simulink model "genpath_user_iface_dc"  (R2022a)
settings: Solver=FixedStepDiscrete  StartTime=0.0  StopTime=inf  RelTol=1e-3  EnableMultiTasking=on
undefined symbols (not defined in the file or in its folder): HW_LOG_VEC_SIZE, HW_LS, HW_RS
libraries: mcbcontrolslib x4, instrumentseriallib x3
settings Model: SimulationMode=accelerator  Creator=61301765  LastModifiedBy=61301765
settings OptimizationCC: DefaultParameterBehavior=Inlined  DefaultUnderspecifiedDataType=single  EnhancedBackFolding=on  PassReuseOutputArgsAs=Individual arguments  ZeroExternalMemoryAtStartup=off  MaxStackSize=64  OptimizeBlockOrder=speed  DifferentSizesBufferReuse=on  OptimizationCustomize=off  EfficientTunableParamExpr=on
settings DebuggingCC: ParameterTunabilityLossMsg=error  UnconnectedInputMsg=warning  UnconnectedOutputMsg=warning  UnconnectedLineMsg=warning
settings HardwareCC: ProdBitPerChar=16  ProdBitPerInt=16  ProdBitPerPointer=32  ProdBitPerSizeT=32  ProdBitPerPtrDiffT=32  ProdLargestAtomicInteger=Integer  ProdLargestAtomicFloat=None  ProdWordSize=16  ProdLongLongMode=on  ProdHWDeviceType=Texas Instruments->C2000
settings SFSimCC: MATLABDynamicMemAlloc=off
settings RTWCC: SystemTargetFile=ert.tlc  TemplateMakefile=ert_default_tmf  Toolchain=Texas Instruments Code Composer Studio (C2000)  DLArmComputeVersion=19.05
settings CodeAppCC: ForceParamTrailComments=on  IgnoreCustomStorageClasses=off  OperatorAnnotations=on  SimulinkDataObjDesc=on  SFDataObjDesc=on  InsertBlockDesc=on
settings ERTTargetCC: ExtModeStaticAllocSize=5000  ERTCustomFileTemplate=example_file_process.tlc

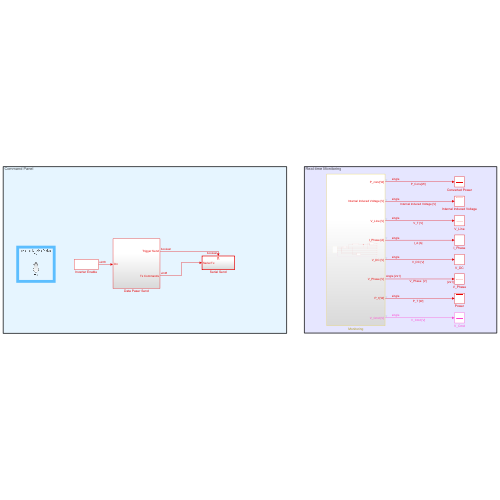
[thumbnail: Simulink's stored preview of the top-level diagram]
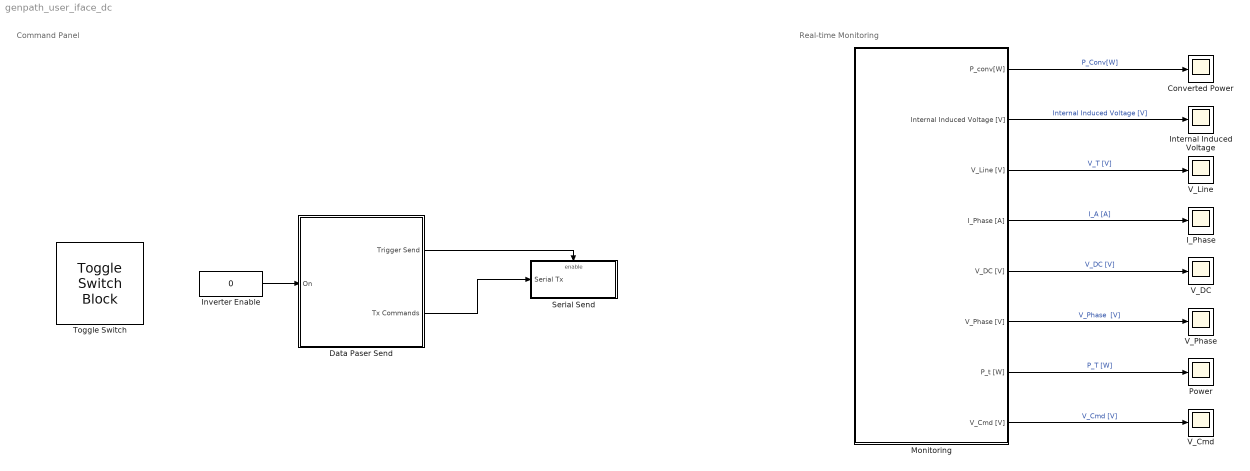
== system genpath_user_iface_dc ==
  note: Real-time Monitoring
  note: Command Panel
  Converted Power : Scope
  Data Paser Send : Subsystem
  I_Phase : Scope
  Internal Induced Voltage : Scope
  Inverter Enable : Constant  Value=0  VectorParams1D=off  OutDataTypeStr=uint8  SampleTime=-1
  Monitoring : Subsystem
  Power : Scope
  Serial Send : Subsystem  TreatAsAtomicUnit=on
  Toggle Switch : ToggleSwitchBlock
      settings: Values={{'Off', 'On'}, [0 1]}
  V_Cmd : Scope
  V_DC : Scope
  V_Line : Scope
  V_Phase : Scope
  wires:
  Data Paser Send/2(Tx Commands) -> Serial Send/1(Serial Tx)
  Data Paser Send/1(Trigger Send) -> Serial Send/Enable
  Inverter Enable/1 -> Data Paser Send/1(On)
  Monitoring/1(P_conv[W]) -> Converted Power/1  "P_Conv[W]"
  Monitoring/3(V_Line [V]) -> V_Line/1  "V_T [V]"
  Monitoring/4(I_Phase [A]) -> I_Phase/1  "I_A [A]"
  Monitoring/5(V_DC [V]) -> V_DC/1  "V_DC [V]"
  Monitoring/6(V_Phase [V]) -> V_Phase/1  "V_Phase  [V]"
  Monitoring/7(P_t [W]) -> Power/1  "P_T [W]"
  Monitoring/2(Internal Induced Voltage [V]) -> Internal Induced Voltage/1  "Internal Induced Voltage [V]"
  Monitoring/8(V_Cmd [V]) -> V_Cmd/1  "V_Cmd [V]"

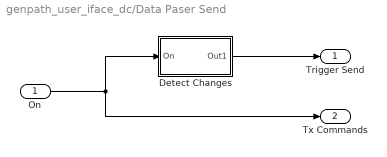
== system genpath_user_iface_dc/Data Paser Send ==
  On : Inport
  Detect Changes : Subsystem
  Trigger Send : Outport  VectorParamsAs1DForOutWhenUnconnected=off
  Tx Commands : Outport  Port=2  VectorParamsAs1DForOutWhenUnconnected=off
  wires:
  Detect Changes/1(Out1) -> Trigger Send/1
  On/1 -> Detect Changes/1(On), Tx Commands/1

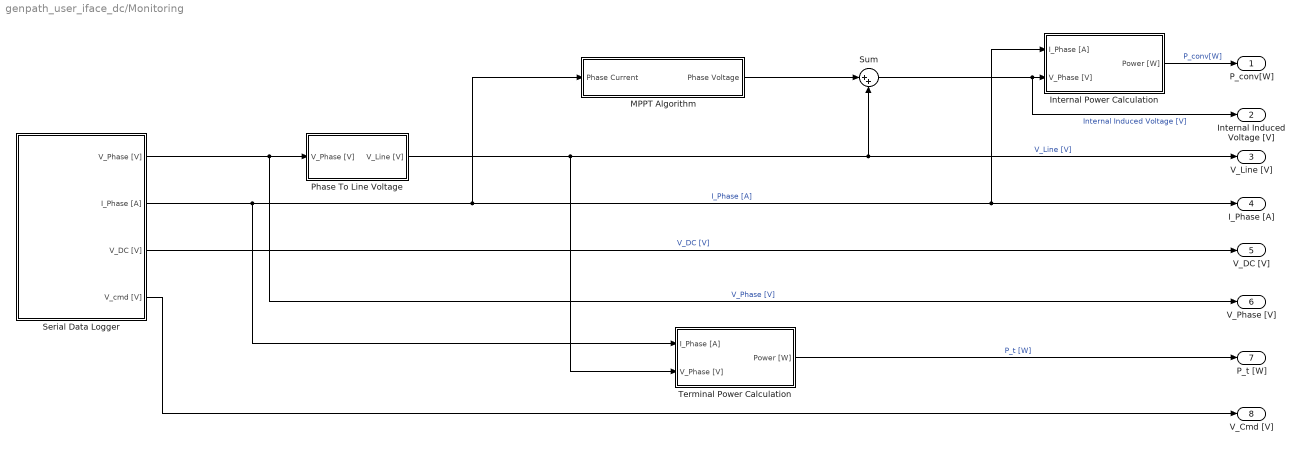
== system genpath_user_iface_dc/Monitoring ==
  Internal Power Calculation : Subsystem
  MPPT Algorithm : Subsystem
  Phase To Line Voltage : Subsystem
  Serial Data Logger : Subsystem
  Sum : Sum  Inputs=|++
  Terminal Power Calculation : Subsystem
  P_conv[W] : Outport
  Internal Induced Voltage [V] : Outport  Port=2
  V_Line [V] : Outport  Port=3
  I_Phase [A] : Outport  Port=4
  V_DC [V] : Outport  Port=5
  V_Phase [V] : Outport  Port=6
  P_t [W] : Outport  Port=7
  V_Cmd [V] : Outport  Port=8
  wires:
  Terminal Power Calculation/1(Power [W]) -> P_t [W]/1  "P_t [W]"
  Serial Data Logger/2(I_Phase [A]) -> Terminal Power Calculation/1(I_Phase [A]), MPPT Algorithm/1(Phase Current), I_Phase [A]/1, Internal Power Calculation/1(I_Phase [A])  "I_Phase [A]"
  Serial Data Logger/1(V_Phase [V]) -> V_Phase [V]/1, Phase To Line Voltage/1(V_Phase [V])  "V_Phase [V]"
  Phase To Line Voltage/1(V_Line [V]) -> Terminal Power Calculation/2(V_Phase [V]), Sum/2, V_Line [V]/1  "V_Line [V]"
  Serial Data Logger/3(V_DC [V]) -> V_DC [V]/1  "V_DC [V]"
  Sum/1 -> Internal Power Calculation/2(V_Phase [V]), Internal Induced Voltage [V]/1  "Internal Induced Voltage [V]"
  Internal Power Calculation/1(Power [W]) -> P_conv[W]/1  "P_conv[W]"
  Serial Data Logger/4(V_cmd [V]) -> V_Cmd [V]/1
  MPPT Algorithm/1(Phase Voltage) -> Sum/1

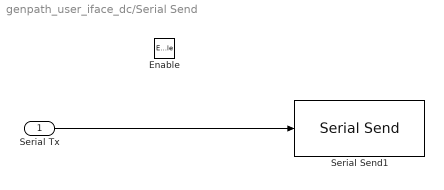
== system genpath_user_iface_dc/Serial Send ==
  Serial Tx : Inport
  Enable : EnablePort
  Serial Send1 : instrumentseriallib/Serial Send  PortSel=COM8  Port=COM8  ComPort=COM8  Header=[ 83 ]  Terminator=Custom terminator  CustomTerminator=[ 69 ]  EnableBlockingMode=on  SimulateUsing=Interpreted execution  BlockInModel=on  aMode=1
      settings: SourceProductBaseCode=OT,IC,MT
  wires:
  Serial Tx/1 -> Serial Send1/1

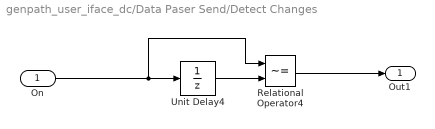
== system genpath_user_iface_dc/Data Paser Send/Detect Changes ==
  On : Inport
  Relational Operator4 : RelationalOperator  Operator=~=  OutDataTypeStr=boolean  InputSameDT=off
  Unit Delay4 : UnitDelay  SampleTime=-1  HasFrameUpgradeWarning=on
  Out1 : Outport  VectorParamsAs1DForOutWhenUnconnected=off
  wires:
  Unit Delay4/1 -> Relational Operator4/2
  On/1 -> Relational Operator4/1, Unit Delay4/1
  Relational Operator4/1 -> Out1/1

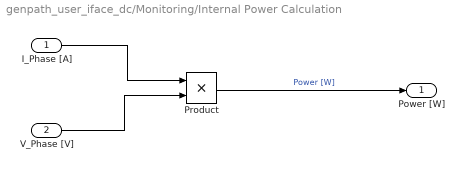
== system genpath_user_iface_dc/Monitoring/Internal Power Calculation ==
  I_Phase [A] : Inport
  V_Phase [V] : Inport  Port=2
  Product : Product
  Power [W] : Outport
  wires:
  Product/1 -> Power [W]/1  "Power [W]"
  V_Phase [V]/1 -> Product/2
  I_Phase [A]/1 -> Product/1

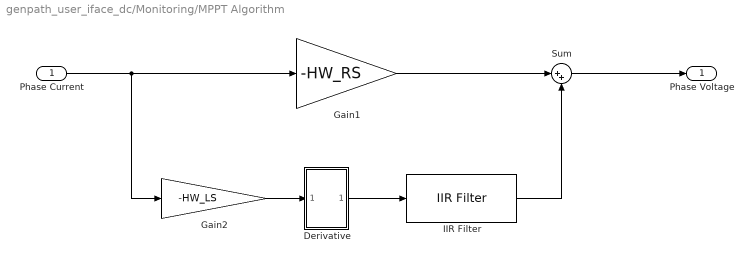
== system genpath_user_iface_dc/Monitoring/MPPT Algorithm ==
  Phase Current : Inport
  Derivative : Subsystem
  Gain1 : Gain  Gain=-HW_RS
  Gain2 : Gain  Gain=-HW_LS
  IIR Filter : mcbcontrolslib/IIR Filter  VariantControl=Low Pass Filter  VariantSelect=Low-pass  Filter_constant=0.2  advancedSettings=on  Ts=100e-6  cutOff_freq=397.8874
      settings: SourceProductBaseCode=MT
  Sum : Sum  Inputs=|++
  Phase Voltage : Outport
  wires:
  Phase Current/1 -> Gain2/1, Gain1/1
  Gain1/1 -> Sum/1
  IIR Filter/1 -> Sum/2
  Gain2/1 -> Derivative/1(In3)
  Derivative/1(Out1) -> IIR Filter/1
  Sum/1 -> Phase Voltage/1

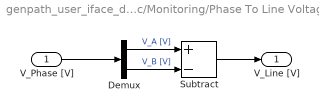
== system genpath_user_iface_dc/Monitoring/Phase To Line Voltage ==
  V_Phase [V] : Inport
  Demux : Demux  Outputs=2
  Subtract : Sum  Inputs=+-
  V_Line [V] : Outport
  wires:
  V_Phase [V]/1 -> Demux/1
  Demux/2 -> Subtract/2  "V_B [V]"
  Demux/1 -> Subtract/1  "V_A [V]"
  Subtract/1 -> V_Line [V]/1

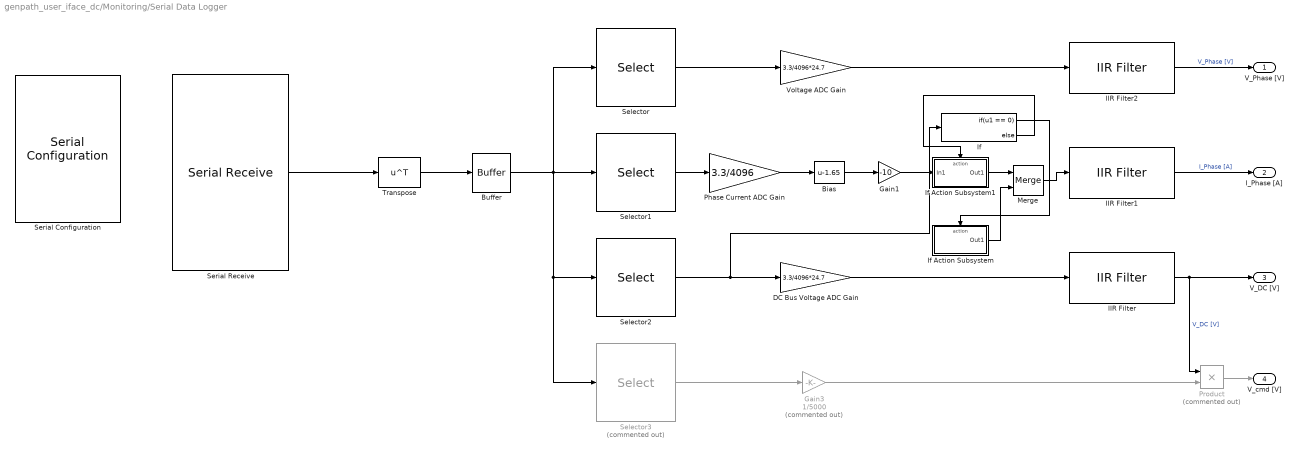
== system genpath_user_iface_dc/Monitoring/Serial Data Logger ==
  Bias : Bias  Bias=-1.65  SaturateOnIntegerOverflow=off
  Buffer : Buffer  N=HW_LOG_VEC_SIZE  OutputFrames=off
  DC Bus Voltage ADC Gain : Gain  Gain=3.3/4096*24.7  OutDataTypeStr=single
  Gain1 : Gain  Gain=-10
  Gain3 : Gain  Commented=on  Gain=1/5000
  IIR Filter : mcbcontrolslib/IIR Filter  VariantControl=Low Pass Filter  VariantSelect=Low-pass  Filter_constant=0.02  advancedSettings=on  Ts=50e-6  cutOff_freq=64.9612
      settings: SourceProductBaseCode=MT
  IIR Filter1 : mcbcontrolslib/IIR Filter  VariantControl=Low Pass Filter  VariantSelect=Low-pass  Filter_constant=0.02  advancedSettings=on  Ts=50e-6  cutOff_freq=64.9612
      settings: SourceProductBaseCode=MT
  IIR Filter2 : mcbcontrolslib/IIR Filter  VariantControl=Low Pass Filter  VariantSelect=Low-pass  Filter_constant=0.5  advancedSettings=on  Ts=50e-6  cutOff_freq=3183.0989
      settings: SourceProductBaseCode=MT
  If : If  IfExpression=u1 == 0
  If Action Subsystem : Subsystem  TreatAsAtomicUnit=on
  If Action Subsystem1 : Subsystem  TreatAsAtomicUnit=on
  Merge : Merge
  Phase Current ADC Gain : Gain  Gain=3.3/4096  OutDataTypeStr=single
  Product : Product  Commented=on
  Selector : Selector  InputPortWidth=HW_LOG_VEC_SIZE  IndexOptions=Index vector (dialog)  Indices=[1 2]  OutputSizes=1
  Selector1 : Selector  InputPortWidth=HW_LOG_VEC_SIZE  IndexOptions=Index vector (dialog)  Indices=[3]  OutputSizes=1
  Selector2 : Selector  InputPortWidth=HW_LOG_VEC_SIZE  IndexOptions=Index vector (dialog)  Indices=4  OutputSizes=1
  Selector3 : Selector  Commented=on  InputPortWidth=HW_LOG_VEC_SIZE  IndexOptions=Index vector (dialog)  Indices=[8 9 10]  OutputSizes=1
  Serial Configuration : instrumentseriallib/Serial Configuration  Priority=-200000  PortSel=COM8  Port=COM8  ComPort=COM8  BaudRate=6250000  DataBits=8  Parity=none  StopBits=1  ByteOrder=little-endian  FlowControl=none  Timeout=1  SimulateUsing=Interpreted execution  BlockInModel=on  aMode=1
      settings: SourceProductBaseCode=OT,IC,MT
  Serial Receive : instrumentseriallib/Serial Receive  PortSel=COM8  Port=COM8  ComPort=COM8  DataType=uint16  SaveDataType=uint8  ToggleHeader=on  Header=[238 238]  ToggleTerminator=on  Terminator=Custom terminator  CustomTerminator=[255 255]  InputFormat=Column major  ToggleDataSize=on  DataSize="[1  1000*HW_LOG_VEC_SIZE]"  EnableBlockingMode=on  ActionDataUnavailable=Output last received value  ActionWhenDataUnavailable=Output last received value  CustomValue=0  SampleTime=0.1  SimulateUsing=Interpreted execution  BlockInModel=on  aMode=1
      settings: SourceProductBaseCode=OT,IC,MT
  Transpose : Math  Operator=transpose  SignedPower=on
  Voltage ADC Gain : Gain  Gain=3.3/4096*24.7  OutDataTypeStr=single
  V_Phase [V] : Outport
  I_Phase [A] : Outport  Port=2
  V_DC [V] : Outport  Port=3
  V_cmd [V] : Outport  Port=4
  wires:
  Serial Receive/1 -> Transpose/1
  Buffer/1 -> Selector2/1, Selector3/1, Selector1/1, Selector/1
  Voltage ADC Gain/1 -> IIR Filter2/1
  Selector/1 -> Voltage ADC Gain/1
  IIR Filter/1 -> Product/1, V_DC [V]/1  "V_DC [V]"
  Selector3/1 -> Gain3/1
  Bias/1 -> Gain1/1
  IIR Filter1/1 -> I_Phase [A]/1  "I_Phase [A]"
  Phase Current ADC Gain/1 -> Bias/1
  Transpose/1 -> Buffer/1
  IIR Filter2/1 -> V_Phase [V]/1  "V_Phase [V]"
  Gain3/1 -> Product/2
  Product/1 -> V_cmd [V]/1
  Selector1/1 -> Phase Current ADC Gain/1
  Selector2/1 -> If/1, DC Bus Voltage ADC Gain/1
  DC Bus Voltage ADC Gain/1 -> IIR Filter/1
  If Action Subsystem/1(Out1) -> Merge/2
  Merge/1 -> IIR Filter1/1
  If/1 -> If Action Subsystem/Action
  If Action Subsystem1/1(Out1) -> Merge/1
  Gain1/1 -> If Action Subsystem1/1(In1)
  If/2 -> If Action Subsystem1/Action

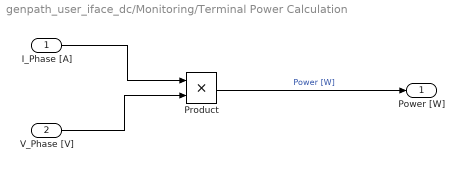
== system genpath_user_iface_dc/Monitoring/Terminal Power Calculation ==
  I_Phase [A] : Inport
  V_Phase [V] : Inport  Port=2
  Product : Product
  Power [W] : Outport
  wires:
  Product/1 -> Power [W]/1  "Power [W]"
  V_Phase [V]/1 -> Product/2
  I_Phase [A]/1 -> Product/1

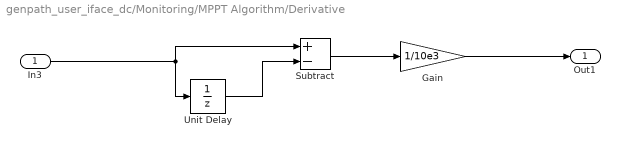
== system genpath_user_iface_dc/Monitoring/MPPT Algorithm/Derivative ==
  In3 : Inport
  Gain : Gain  Gain=1/10e3
  Subtract : Sum  Inputs=+-
  Unit Delay : UnitDelay  SampleTime=-1  HasFrameUpgradeWarning=on
  Out1 : Outport
  wires:
  In3/1 -> Unit Delay/1, Subtract/1
  Unit Delay/1 -> Subtract/2
  Subtract/1 -> Gain/1
  Gain/1 -> Out1/1

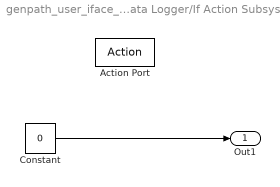
== system genpath_user_iface_dc/Monitoring/Serial Data Logger/If Action Subsystem ==
  Action Port : ActionPort  ActionPortLabel=if(u1 == 0)
  Constant : Constant  Value=0  OutDataTypeStr=Inherit: Inherit via back propagation
  Out1 : Outport
  wires:
  Constant/1 -> Out1/1

== system genpath_user_iface_dc/Monitoring/Serial Data Logger/If Action Subsystem1 ==
  In1 : Inport
  Action Port : ActionPort  ActionPortLabel=else
  Out1 : Outport
  wires:
  In1/1 -> Out1/1
